simulink model "HW2_Q.3_sysmokh"  (R2017b)
settings: Solver=VariableStepAuto  StartTime=0.0  StopTime=0.9  RelTol=1e-3
undefined symbols (not defined in the file or in its folder): Newton, Raphson
libraries: dspmlti4 x2, dspsrcs4 x1
settings Model: Creator=ali  LastModifiedBy=ali

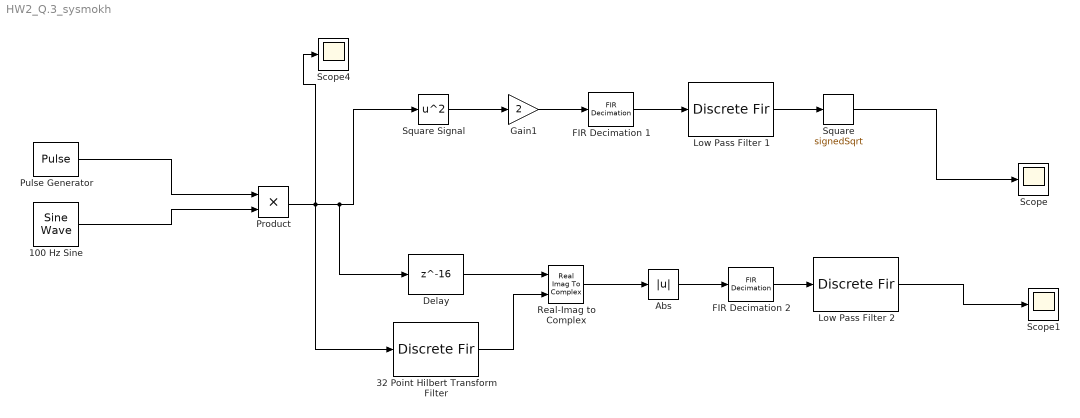
== system HW2_Q.3_sysmokh ==
  100 Hz Sine : dspsrcs4/Sine Wave  Amplitude=1  Frequency=100  Phase=0  SampleMode=Discrete  OutComplex=Real  CompMethod=Trigonometric fcn  TableSize=Speed  SampleTime=1/22050  SamplesPerFrame=1  ResetState=Restart at time zero  OutputFrames=on  dataType=double  wordLen=16  udDataType=sfix(16)  fracBitsMode=Best precision  numFracBits=15  OutDataTypeStr=double  LastOutDataTypeStr=double
  32 Point Hilbert Transform Filter : DiscreteFir  Coefficients=firpm(32, [0.1 0.9], [1 1], 'hilbert')  AccumDataTypeStr=Inherit: Same as product output
  Abs : Abs
  Delay : Delay  DelayLength=16  InitialCondition=0
  FIR Decimation 1 : dspmlti4/FIR Decimation  FilterSource=Dialog parameters  h=[1 1]  D=15  filtStruct=Direct form  FilterObject=Hm_firdecim  framing=Allow multirate processing  inputOffset=0  outputBufInitCond=0  roundingMode=Floor  overflowMode=off  firstCoeffDataTypeStr=Inherit: Same word length as input  firstCoeffMin=[]  firstCoeffMax=[]  firstCoeffLastDataTypeStr=Inherit: Same word length as input  outputMin=[]  outputMax=[]
  FIR Decimation 2 : dspmlti4/FIR Decimation  FilterSource=Dialog parameters  h=[1 1]  D=15  filtStruct=Direct form  FilterObject=Hm_firdecim  framing=Allow multirate processing  inputOffset=0  outputBufInitCond=0  roundingMode=Floor  overflowMode=off  firstCoeffDataTypeStr=Inherit: Same word length as input  firstCoeffMin=[]  firstCoeffMax=[]  firstCoeffLastDataTypeStr=Inherit: Same word length as input  outputMin=[]  outputMax=[]
  Gain1 : Gain  Gain=2
  Low Pass Filter 1 : DiscreteFir  Coefficients=firpm(20, [0 0.03 0.1 1], [1 1 0 0])  AccumDataTypeStr=Inherit: Same as product output
  Low Pass Filter 2 : DiscreteFir  Coefficients=firpm(20, [0 0.03 0.1 1], [1 1 0 0])  AccumDataTypeStr=Inherit: Same as product output
  Product : Product  RndMeth=Zero
  Pulse Generator : DiscretePulseGenerator  Amplitude=0.5  Period=7000  PulseWidth=4000  SampleTime=1/22050
  Real-Imag to Complex : RealImagToComplex
  Scope : Scope
  Scope1 : Scope
  Scope4 : Scope
  "Square " : Sqrt  Operator=signedSqrt  AlgorithmType=Newton-Raphson  SaturateOnIntegerOverflow=on
  Square Signal : Math  Operator=square  SaturateOnIntegerOverflow=on
  wires:
  Pulse Generator/1 -> Product/1
  100 Hz Sine/1 -> Product/2
  Product/1 -> Scope4/1, 32 Point Hilbert Transform Filter/1, Delay/1, Square Signal/1
  Square Signal/1 -> Gain1/1
  Gain1/1 -> FIR Decimation 1/1
  FIR Decimation 1/1 -> Low Pass Filter 1/1
  Low Pass Filter 1/1 -> "Square "/1
  "Square "/1 -> Scope/1
  Low Pass Filter 2/1 -> Scope1/1
  FIR Decimation 2/1 -> Low Pass Filter 2/1
  Abs/1 -> FIR Decimation 2/1
  Real-Imag to Complex/1 -> Abs/1
  Delay/1 -> Real-Imag to Complex/1
  32 Point Hilbert Transform Filter/1 -> Real-Imag to Complex/2
